simulink library "hapsrav_library"  (R2017a)
settings: Solver=VariableStepAuto  StartTime=0.0  StopTime=10.0  RelTol=1e-3
values from neighbouring files (symbols this model uses):
  absorb_h = 0:100:40000    [EnergySim.m]
  Adisk = pi * v.R_prop^2    [EnergySim.m]
  alpha_h = absorb_h    [EnergySim.m]
  aoa_data = zeros(n_cl, n)    [EnergySim.m]
  cl_bp = linspace(min_cl, max_cl,n_cl)    [EnergySim.m]
  D = [1       -.0065      288.15          0                   101325 ... (first row only)    [EnergySim.m]    (also in msn_params.m = sqrt((from_x - to_x)^2 + (from_y - to_y)^2); solar_vector.m = time.day + ut_time)
  d2r = pi / 180    (= 0.0174532925199)    [EnergySim.m]    (also in example1.m; example2.m; example3.m; example4.m)
  d_init = sqrt(dx*dx + dy*dy)    [EnergySim.m]    (also in msn_init.m)
  dchi0 = atan2(sin(dchi0), cos(dchi0))    [EnergySim.m]    (also in msn_init.m)
  dT = 0.5    [EnergySim.m]
  dT_fixed = 0.5    [EnergySim.m]
  dT_trig = 30    [EnergySim.m]
  earth_rho = 6378137.0    (= 6378137)    [EnergySim.m]
  fp = solarFP(p.orbit_rho, p.min_axis, p.orbit_dir, ic.x_ctr, ic.y_ctr, sun_az_0)    [EnergySim.m]    (also in load_fp.m = gid_tc(msn_idx).fp; solarFP.m = [1	6	2	nul eul 0	0	0	0	1	0)
  fp_coords = [x_entry y_entry]    [msn_params.m]
  fp_courses = [chi_adj nxt_chi dchi]    [msn_params.m]
  g = 9.80665    [EnergySim.m]
  Gsolar = 1367    [EnergySim.m]
  k = k+1    (= 5)    [EnergySim.m]
  K = D(:,2)    [EnergySim.m]
  lat_init = ic.lat_init_deg * obj.d2r    [EnergySim.m]
  M = time.month    [solar_vector.m]
  max_cl = max(cl_data(:))    [EnergySim.m]
  min_cl = min(cl_data(:))    [EnergySim.m]
  ND2 = load(fullfile(pwd,'nd2_data.mat'))    [EnergySim.m]    (also in nd2_data.mat = [0.0999999999999 0.200000000001 0.3 0.4 0.499999999998 0.700)
  next_init = fp(init_wp, 3)    [EnergySim.m]    (also in msn_init.m)
  pE_init = ic.pE_init    [EnergySim.m]
  pN_init = ic.pN_init    [EnergySim.m]
  r2d = 180 / pi    (= 57.2957795131)    [EnergySim.m]    (also in example1.m; example2.m; example3.m; example4.m)
  rho_SL = 1.225    [EnergySim.m]
  S = 110.4    [EnergySim.m]
  thr_lo_lim = 0.0    (= 0)    [EnergySim.m]
  time_init = struct('year', time.year, 'month', time.month,                  'day', time.day, 'hour', time.hour, 'min', time.min,                  'UTC', time.UTC)    [EnergySim.m]
  to_init = fp(init_wp, 1)    [EnergySim.m]    (also in msn_init.m)
  vgnd_init = sqrt(Vg)    [EnergySim.m]
  vtas_init = veas_init * sqrt(rho_sl/rho_alt)    [EnergySim.m]
  w_alt = 2.0 * w_alt    [EnergySim.m]
  w_xtrack = 2.0 * w_xtrack    [EnergySim.m]
undefined symbols (not defined in the file or in its folder): alpha, alpha_bp, alpha_circ, alt0_rate_init, alt_bp, alt_cmd_mode, alt_init, alt_lim_h, alt_lim_l, alt_rt_lim_periodic, cd_data, charge_eff, chi0_rate_init, chi_cmd_mode, chi_inf, chi_init, cl_data, discharge_eff, DiscIntNeverNeededParam, E_batt_max, E_init, Earth, enableFuzzyLogic, entry_init, epsln, epsln_circ, exit_init, f8_azimuth_offset, fig_eight_time, fp0, fp_coords0, fp_courses0, gamma_lim, hold_time, k_c, K_circ, lat_init_deg, lon_init_deg, max_alpha_bp, max_alt_bp, min_alpha_bp, min_alt_bp, min_axis, motor_eff, mppt_eff, num_motors, orb_dir_init, orb_len_init, orbit_dir, orbit_rho, P_acc, panel_eff, panel_vecs, phi_0, phi_lim, phi_lim_alt, phi_lim_alt_max, phi_lim_alt_min, phi_rt_lim, prop_eff_scale ... (+39)
libraries: simulink x59, hapsrav_library x9, fuzblock x3, atmospheric_library x1, aerolibtransform2 x1
(part 4 of 6)

== system hapsrav_library/hapsrav_main/Kinematic 6DOF/Aero/CL vs AoA/alpha RLUT ==
  alt : Inport
  CL : Inport  Port=2
  0 <= Alt < 20574 : Subsystem  Commented=on  TreatAsAtomicUnit=on
  0 <= Alt <= 24575 : Saturate  UpperLimit=max_alt_bp  LowerLimit=min_alt_bp
  0.73 <= CL <= 1.43 : Saturate  UpperLimit=max_cl  LowerLimit=min_cl
  20574 <= Alt < 21908 : Subsystem  Commented=on  TreatAsAtomicUnit=on
  21908 <= Alt < 23241 : Subsystem  Commented=on  TreatAsAtomicUnit=on
  23241 <= Alt < 24575 : Subsystem  Commented=on  TreatAsAtomicUnit=on
  AoA LUT : Lookup_n-D  BreakpointsForDimension1=cl_bp  BreakpointsForDimension2=alt_bp  IndexSearchMethod=Linear search  BeginIndexSearchUsingPreviousIndexResult=on  Table=aoa_data  ExtrapMethod=Clip  RemoveProtectionInput=on  UseLastTableValue=on  InternalRulePriority=Speed  RndMeth=Simplest  InputSameDT=on
  From{,1..2,4,6} (5 alike) : From  Commented=on  GotoTag=alt
  From{3,5,7..8} (4 alike) : From  Commented=on  GotoTag=CL
  Interval Test : simulink/Logic and Bit Operations/Interval Test  Commented=on  IntervalClosedRight=off  uplimit=alt_bp(2)  IntervalClosedLeft=on  lowlimit=alt_bp(1)  OutDataTypeStr=boolean
  Interval Test1 : simulink/Logic and Bit Operations/Interval Test  Commented=on  IntervalClosedRight=off  uplimit=alt_bp(3)  IntervalClosedLeft=on  lowlimit=alt_bp(2)  OutDataTypeStr=boolean
  Interval Test2 : simulink/Logic and Bit Operations/Interval Test  Commented=on  IntervalClosedRight=off  uplimit=alt_bp(4)  IntervalClosedLeft=on  lowlimit=alt_bp(3)  OutDataTypeStr=boolean
  Interval Test3 : simulink/Logic and Bit Operations/Interval Test  Commented=on  IntervalClosedRight=on  uplimit=alt_bp(5)  IntervalClosedLeft=on  lowlimit=alt_bp(4)  OutDataTypeStr=boolean
  Merge : Merge  Commented=on  Inputs=4
  alpha_rad : Outport
  wires:
  0.73 <= CL <= 1.43/1 -> [CL]
  0 <= Alt <= 24575/1 -> [alt]
  From1/1 -> Interval Test/1, Interval Test3/1, Interval Test2/1, Interval Test1/1
  20574 <= Alt < 21908/1(alpha) -> Merge/2
  alt/1 -> 0 <= Alt <= 24575/1
  From8/1 -> 0 <= Alt < 20574/1(CL)
  From3/1 -> 20574 <= Alt < 21908/1(CL)
  0 <= Alt < 20574/1(alpha) -> Merge/1
  Interval Test3/1 -> 23241 <= Alt < 24575/Enable
  From2/1 -> 20574 <= Alt < 21908/2(alt)
  CL/1 -> 0.73 <= CL <= 1.43/1
  Interval Test2/1 -> 21908 <= Alt < 23241/Enable
  23241 <= Alt < 24575/1(alpha) -> Merge/4
  From7/1 -> 23241 <= Alt < 24575/1(CL)
  From4/1 -> 21908 <= Alt < 23241/2(alt)
  From5/1 -> 21908 <= Alt < 23241/1(CL)
  From6/1 -> 23241 <= Alt < 24575/2(alt)
  Interval Test/1 -> 0 <= Alt < 20574/Enable
  21908 <= Alt < 23241/1(alpha) -> Merge/3
  From/1 -> 0 <= Alt < 20574/2(alt)
  Interval Test1/1 -> 20574 <= Alt < 21908/Enable
  [CL] -> AoA LUT/1
  [alt] -> AoA LUT/2
  AoA LUT/1 -> alpha_rad/1

== system hapsrav_library/hapsrav_main/Kinematic 6DOF/Navigation/Flat Earth to LLA/Radii of Curvature ==
  lat_rad : Inport
  h : Inport  Port=2
  Divide : Product  Inputs=*/
  Divide1 : Product  Inputs=**
  Divide2 : Product  Inputs=*/
  Gain1 : Gain  Gain=wgs84.e2
  Math Function : Math  Operator=square  SaturateOnIntegerOverflow=on
  Sqrt : Sqrt  SaturateOnIntegerOverflow=on
  Sum : Sum  Inputs=|+-
  Sum1 : Sum  Inputs=+-|
  Sum2 : Sum  Inputs=|++
  Sum3 : Sum  Inputs=|++
  Trigonometric Function : Trigonometry
  href3 : Constant
  href4 : Constant  Value=wgs84.a
  href5 : Constant  Value=wgs84.e2
  href6 : Constant
  R_N : Outport
  R_M : Outport  Port=2
  wires:
  Sum1/1 -> Divide1/2
  href3/1 -> Sum/1
  Gain1/1 -> Sum/2
  Math Function/1 -> Gain1/1
  Sqrt/1 -> [den_0p5]
  href4/1 -> Divide/1
  href6/1 -> Sum1/1
  href5/1 -> Sum1/2
  Divide/1 -> Divide1/1, Sum2/1  "Prime Vert ROC"
  [den_0p5] -> Divide/2
  [den] -> Divide2/2
  Divide1/1 -> Divide2/1
  lat_rad/1 -> Trigonometric Function/1
  Trigonometric Function/1 -> Math Function/1
  Sum/1 -> Sqrt/1, [den]
  h/1 -> [h]
  Sum2/1 -> R_N/1
  [h] -> Sum2/2
  Divide2/1 -> Sum3/1  "Meridian ROC"
  Sum3/1 -> R_M/1
  [h] -> Sum3/2

== system hapsrav_library/hapsrav_main/Kinematic 6DOF/Power Model/Battery and Potential Management/Climb Rate ==
  ClimbMode : Inport
  P_el_out : Inport  Port=2
  P_el_net_cruise : Inport  Port=3
  P_el_net : Inport  Port=4
  Constant4 : Constant  Value=0
  Constant7 : Constant  Value=P_acc*0.001
  Delay1 : Delay  DelayLength=1
  Gain1 : Gain  Gain=-1
  Gain2 : Gain  Gain=1/M
  Gain3 : Gain  Gain=1/g
  Multiport Switch1 : MultiPortSwitch  DataPortOrder=Specify indices  DataPortIndices={-2, -1, 0, 1}
  PID Controller : simulink/Continuous/PID Controller  Controller=PID  TimeDomain=Discrete-time  SampleTime=-1  IntegratorMethod=Forward Euler  FilterMethod=Forward Euler  Form=Parallel  UseFilter=off  ControllerParametersSource=internal  P=1.1  I=0.001  D=0  N=0.1  InitialConditionSource=internal  InitialConditionForIntegrator=0  InitialConditionForFilter=0  ExternalReset=either  LimitOutput=off  UpperSaturationLimit=inf  LowerSaturationLimit=-inf  LinearizeAsGain=off  AntiWindupMode=none  Kb=1  TrackingMode=off  Kt=1  PParamMin=[]  PParamMax=[]  IParamMin=[]  IParamMax=[]  DParamMin=[]  DParamMax=[]  NParamMin=[]  NParamMax=[]  KbParamMin=[]  KbParamMax=[]  KtParamMin=[]  KtParamMax=[]  POutMin=[]  POutMax=[]  IOutMin=[]  IOutMax=[]  DOutMin=[]  DOutMax=[]  NOutMin=[]  NOutMax=[]  KbOutMin=[]  KbOutMax=[]  KtOutMin=[]  KtOutMax=[]  IntegratorOutMin=[]  IntegratorOutMax=[]  FilterOutMin=[]  FilterOutMax=[]  SumOutMin=[]  SumOutMax=[]  SumI1OutMin=[]  SumI1OutMax=[]  SumI2OutMin=[]  SumI2OutMax=[]  SumI3OutMin=[]  SumI3OutMax=[]  SumDOutMin=[]  SumDOutMax=[]  SaturationOutMin=[]  SaturationOutMax=[]  IntegratorContinuousStateAttributes=''  IntegratorStateMustResolveToSignalObject=off  IntegratorRTWStateStorageClass=Auto  FilterContinuousStateAttributes=''  FilterStateMustResolveToSignalObject=off  FilterRTWStateStorageClass=Auto  DifferentiatorICPrevScaledInput=0  DifferentiatorOutMin=[]  DifferentiatorOutMax=[]  InitialConditionSetting=State (most efficient)
  PID Controller1 : simulink/Continuous/PID Controller  Controller=PID  TimeDomain=Discrete-time  SampleTime=-1  IntegratorMethod=Forward Euler  FilterMethod=Forward Euler  Form=Parallel  UseFilter=off  ControllerParametersSource=internal  P=2.5  I=0.001  D=0  N=0.1  InitialConditionSource=internal  InitialConditionForIntegrator=0  InitialConditionForFilter=0  ExternalReset=either  LimitOutput=off  UpperSaturationLimit=inf  LowerSaturationLimit=-inf  LinearizeAsGain=off  AntiWindupMode=none  Kb=1  TrackingMode=off  Kt=1  PParamMin=[]  PParamMax=[]  IParamMin=[]  IParamMax=[]  DParamMin=[]  DParamMax=[]  NParamMin=[]  NParamMax=[]  KbParamMin=[]  KbParamMax=[]  KtParamMin=[]  KtParamMax=[]  POutMin=[]  POutMax=[]  IOutMin=[]  IOutMax=[]  DOutMin=[]  DOutMax=[]  NOutMin=[]  NOutMax=[]  KbOutMin=[]  KbOutMax=[]  KtOutMin=[]  KtOutMax=[]  IntegratorOutMin=[]  IntegratorOutMax=[]  FilterOutMin=[]  FilterOutMax=[]  SumOutMin=[]  SumOutMax=[]  SumI1OutMin=[]  SumI1OutMax=[]  SumI2OutMin=[]  SumI2OutMax=[]  SumI3OutMin=[]  SumI3OutMax=[]  SumDOutMin=[]  SumDOutMax=[]  SaturationOutMin=[]  SaturationOutMax=[]  IntegratorContinuousStateAttributes=''  IntegratorStateMustResolveToSignalObject=off  IntegratorRTWStateStorageClass=Auto  FilterContinuousStateAttributes=''  FilterStateMustResolveToSignalObject=off  FilterRTWStateStorageClass=Auto  DifferentiatorICPrevScaledInput=0  DifferentiatorOutMin=[]  DifferentiatorOutMax=[]  InitialConditionSetting=State (most efficient)
  Saturation : Saturate  UpperLimit=2.08  LowerLimit=-2.08
  Sum3 : Sum  Inputs=|+-
  kW to W : Gain  Gain=1000
  powered_climb_rt : Outport
  wires:
  PID Controller1/1 -> Multiport Switch1/2
  Constant7/1 -> Sum3/2
  P_el_out/1 -> Sum3/1
  Gain1/1 -> PID Controller1/1
  Sum3/1 -> Gain1/1
  PID Controller/1 -> Multiport Switch1/3
  P_el_net_cruise/1 -> PID Controller/1
  Saturation/1 -> powered_climb_rt/1
  Constant4/1 -> Multiport Switch1/4
  P_el_net/1 -> Multiport Switch1/5
  Multiport Switch1/1 -> Delay1/1
  ClimbMode/1 -> Multiport Switch1/1, PID Controller/2, PID Controller1/2
  Gain3/1 -> Saturation/1  "Max Clmb Rt"
  kW to W/1 -> Gain2/1
  Gain2/1 -> Gain3/1
  Delay1/1 -> kW to W/1

== system hapsrav_library/hapsrav_main/Kinematic 6DOF/Power Model/Electric Power In/atmos_absorb_adj ==
  sun_zth : Inport
  altitude : Inport  Port=2
  Trigger : TriggerPort  TriggerType=either  VariantControl=Variant  InitialTriggerSignalState=positive
  Constant : Constant  Value=earth_rho
  Constant1 : Constant  Value=alpha_h
  Constant2 : Constant  Value=absorb_h
  Gain : Gain  Gain=0.001
  Gain1 : Gain  Gain=0.001
  atmospheric adjustment : MATLAB Function  TreatAsAtomicUnit=on
  atmos_adj : Outport
  wires:
  altitude/1 -> Gain/1
  sun_zth/1 -> atmospheric adjustment/2(zth)
  Constant/1 -> Gain1/1
  Gain/1 -> atmospheric adjustment/1(h)  "h (km)"
  Gain1/1 -> atmospheric adjustment/3(earth_rho)
  Constant1/1 -> atmospheric adjustment/4(alpha_h)
  Constant2/1 -> atmospheric adjustment/5(absorb_h)
  atmospheric adjustment/1(rel_power) -> atmos_adj/1

== system hapsrav_library/hapsrav_main/Kinematic 6DOF/Power Model/Electric Power In/projected area ==
  yaw : Inport
  pitch : Inport  Port=2
  roll : Inport  Port=3
  sun : Inport  Port=4
  Projected area : MATLAB Function  TreatAsAtomicUnit=on
  panel directions : Constant  Value=panel_vecs
  projected_area : Outport
  wires:
  yaw/1 -> Projected area/1(y)
  roll/1 -> Projected area/3(r)
  pitch/1 -> Projected area/2(p)
  Projected area/1(proj_area) -> projected_area/1
  panel directions/1 -> Projected area/4(panel_vecs)
  sun/1 -> Projected area/5(sun_vector)

== system hapsrav_library/hapsrav_main/Kinematic 6DOF/Power Model/Electric Power In/solar_dist_adj ==
  jd : Inport
  Trigger : TriggerPort  TriggerType=either  VariantControl=Variant  InitialTriggerSignalState=positive
  2*pi/365.1 : Gain  Gain=0.034
  2*pi/365.25 : Gain  Gain=2*pi/365.25
  Add : Sum
  Constant : Constant
  Cos : Trigonometry  Operator=cos
  dist_adj : Outport
  wires:
  Constant/1 -> Add/1
  2*pi/365.1/1 -> Add/2
  Cos/1 -> 2*pi/365.1/1
  jd/1 -> 2*pi/365.25/1
  2*pi/365.25/1 -> Cos/1
  Add/1 -> dist_adj/1

== system hapsrav_library/hapsrav_main/Kinematic 6DOF/Power Model/Electric Power In/solar_vec_ned ==
  az : Inport
  zth : Inport  Port=2
  Trigger : TriggerPort  TriggerType=either  VariantControl=Variant  InitialTriggerSignalState=positive
  Gain1 : Gain  Gain=d2r
  Gain2 : Gain  Gain=d2r
  Gain3 : Gain  Gain=-1
  Gain4 : Gain  Gain=-1
  Mux1 : Mux  Inputs=3
  Mux2 : Mux  Inputs=3
  Subtract : Sum  Inputs=-+
  Trigonometric Function : Trigonometry
  Trigonometric Function1 : Trigonometry  Operator=cos
  Trigonometric Function2 : Trigonometry
  Trigonometric Function3 : Trigonometry  Operator=cos
  clip when below horizon : Switch  Criteria=u2 > Threshold
  complement : Constant  Value=pi/2
  complement1 : Constant  Value=0
  complement2 : Constant  Value=0
  complement3 : Constant  Value=0
  pow_calc1 : Product
  pow_calc2 : Product
  sun_ned : Outport
  wires:
  Gain2/1 -> Subtract/1
  Gain4/1 -> Mux1/2
  complement3/1 -> Mux2/3
  [c_el] -> pow_calc1/2
  zth/1 -> Gain2/1
  az/1 -> Gain1/1
  Mux2/1 -> clip when below horizon/3
  Gain3/1 -> Mux1/1
  Subtract/1 -> clip when below horizon/2, Trigonometric Function3/1, Trigonometric Function2/1  "el"
  Trigonometric Function1/1 -> [c_az]
  complement2/1 -> Mux2/2
  Trigonometric Function2/1 -> [s_el]
  [s_az] -> pow_calc2/1
  [c_el] -> pow_calc2/2
  [s_el] -> Mux1/3
  complement1/1 -> Mux2/1
  Trigonometric Function3/1 -> [c_el]
  Gain1/1 -> Trigonometric Function1/1, Trigonometric Function/1
  [c_az] -> pow_calc1/1
  clip when below horizon/1 -> sun_ned/1
  Mux1/1 -> clip when below horizon/1
  complement/1 -> Subtract/2
  Trigonometric Function/1 -> [s_az]
  pow_calc2/1 -> Gain4/1
  pow_calc1/1 -> Gain3/1

== system hapsrav_library/hapsrav_main/Kinematic 6DOF/Power Model/Electric Power Out/prop_eff (theoretical max from actuator disk theory, scaled by coeff < 1) (http:////web.mit.edu//16.unified//www//FALL//thermodynamics//notes//node86.html) ==
  thrust : Inport
  qbar : Inport  Port=2
  Add : Sum
  Add1 : Sum
  Constant : Constant
  Constant1 : Constant
  Constant2 : Constant  Value=2
  Divide1 : Product  Inputs=*/
  Divide2 : Product  Inputs=*/
  Sqrt : Sqrt  SaturateOnIntegerOverflow=on
  disk_area : Gain  Gain=Adisk
  num_motors : Gain  Gain=num_motors
  scale_by_const : Gain  Gain=prop_eff_scale
  prop_eff : Outport
  wires:
  Constant2/1 -> Divide2/1
  Divide1/1 -> Add/2
  Divide2/1 -> scale_by_const/1  "theoretical max"
  Constant/1 -> Add/1
  Add/1 -> Sqrt/1
  Add1/1 -> Divide2/2
  Sqrt/1 -> Add1/2
  Constant1/1 -> Add1/1
  scale_by_const/1 -> prop_eff/1
  thrust/1 -> Divide1/1
  disk_area/1 -> num_motors/1
  num_motors/1 -> Divide1/2
  qbar/1 -> disk_area/1

== system hapsrav_library/hapsrav_main/Kinematic 6DOF/Selectable Modes/Trajectory_Optimization/Altitude ==
  altRt_cmd : Inport
  max_clmb_rt : Inport  Port=2
  max_desc_rt : Inport  Port=3
  alt0 : Inport  Port=4
  altRt0 : Inport  Port=5
  idleDesc : Inport  Port=6
  Delay1 : Delay  DelayLength=1  InitialConditionSource=Input port
      settings: InputPortMap=u0,p4
  Discrete-Time Integrator : DiscreteIntegrator  IntegratorMethod=Integration: Trapezoidal  InitialConditionSource=external  InitialConditionSetting=State (most efficient)  SampleTime=-1  ICPrevOutput=DiscIntNeverNeededParam  ICPrevScaledInput=DiscIntNeverNeededParam
  Mux : Mux  Inputs=2
  Scope : Scope
  Sum : Sum  Inputs=|+-
  alt_rate : Subsystem
  u_wn^2 : Gain  Gain=w_alt * w_alt
  alt : Outport
  d1alt : Outport  Port=2
  wires:
  [alt_rate] -> Mux/1
  [cmd] -> Mux/2
  [cmd] -> Sum/1
  altRt_cmd/1 -> [cmd]
  Mux/1 -> Scope/1
  [alt_rate] -> d1alt/1
  max_desc_rt/1 -> alt_rate/2(max_desc_rt)
  idleDesc/1 -> alt_rate/5(idleDesc)
  alt0/1 -> Discrete-Time Integrator/2
  Delay1/1 -> Sum/2
  alt_rate/1(d1alt) -> Discrete-Time Integrator/1, [alt_rate], Delay1/1
  Discrete-Time Integrator/1 -> alt/1
  Sum/1 -> u_wn^2/1
  max_clmb_rt/1 -> alt_rate/1(max_clmb_rt)
  u_wn^2/1 -> alt_rate/3(d2alt)
  altRt0/1 -> [altRt0]
  [altRt0] -> Delay1/2
  [altRt0] -> alt_rate/4(altRt0)

== system hapsrav_library/hapsrav_main/Kinematic 6DOF/Selectable Modes/Trajectory_Optimization/Lat Cmd Filter ==
  roll cmd : Inport
  roll0 : Inport  Port=2
  1/tau : Gain  Gain=0.1
  Delay1 : Delay  DelayLength=1  InitialConditionSource=Input port
      settings: InputPortMap=u0,p4
  Discrete-Time Integrator : DiscreteIntegrator  IntegratorMethod=Integration: Trapezoidal  InitialConditionSource=external  InitialConditionSetting=State (most efficient)  SampleTime=-1  ICPrevOutput=DiscIntNeverNeededParam  ICPrevScaledInput=DiscIntNeverNeededParam
  Sum : Sum  Inputs=|+-
  filt roll cmd : Outport
  wires:
  [roll0] -> Discrete-Time Integrator/2
  [roll0] -> Delay1/2
  roll0/1 -> [roll0]
  Delay1/1 -> Sum/2
  roll cmd/1 -> Sum/1
  Discrete-Time Integrator/1 -> filt roll cmd/1, Delay1/1
  Sum/1 -> 1/tau/1
  1/tau/1 -> Discrete-Time Integrator/1

== system hapsrav_library/hapsrav_main/Kinematic 6DOF/Selectable Modes/Trajectory_Optimization/Roll ==
  filtRollcmd : Inport
  roll0 : Inport  Port=2
  alt : Inport  Port=3
  Vg : Inport  Port=4
  chi0 : Inport  Port=5
  Delay1 : Delay  DelayLength=1  InitialConditionSource=Input port
      settings: InputPortMap=u0,p4
  Saturation Dynamic : simulink/Discontinuities/Saturation Dynamic  OutMin=[]  OutMax=[]  OutDataTypeStr=Inherit: Same as second input  OutDataType=fixdt(1, 16)  OutScaling=2^-10  DoSatur=off
  Sum : Sum  Inputs=|+-
  a : Gain  Gain=-1
  phi_lim LUT : Lookup_n-D  NumberOfTableDimensions=1  BreakpointsForDimension1=phi_lim_alt  Table=phi_lim  ExtrapMethod=Clip  DiagnosticForOutOfRangeInput=Error  RemoveProtectionInput=on  UseLastTableValue=on  InternalRulePriority=Speed  RndMeth=Simplest  InputSameDT=on
  phi_rt_lim LUT : Lookup_n-D  NumberOfTableDimensions=1  BreakpointsForDimension1=phi_lim_alt  Table=phi_rt_lim  ExtrapMethod=Clip  DiagnosticForOutOfRangeInput=Error  RemoveProtectionInput=on  UseLastTableValue=on  InternalRulePriority=Speed  RndMeth=Simplest  InputSameDT=on
  roll_angle : Subsystem
  u_wn^2 : Gain  Gain=w_xtrack * w_xtrack
  roll : Outport
  chi : Outport  Port=2
  wires:
  roll_angle/1(chi) -> chi/1
  chi0/1 -> roll_angle/5(chi0)
  Vg/1 -> roll_angle/4(Vg)
  u_wn^2/1 -> Saturation Dynamic/2
  filtRollcmd/1 -> Sum/1
  Sum/1 -> u_wn^2/1
  roll_angle/2(roll) -> Delay1/1, roll/1
  Delay1/1 -> Sum/2
  roll0/1 -> roll_angle/3(roll0), [roll0]
  [roll0] -> Delay1/2
  phi_lim LUT/1 -> [phi_lim]
  phi_rt_lim LUT/1 -> [phi_rt_lim]
  alt/1 -> phi_rt_lim LUT/1, phi_lim LUT/1
  [phi_lim] -> roll_angle/1(roll_lim)
  [phi_rt_lim] -> Saturation Dynamic/1
  [phi_rt_lim] -> a/1
  a/1 -> Saturation Dynamic/3
  Saturation Dynamic/1 -> roll_angle/2(d1roll)

== system hapsrav_library/hapsrav_main/Kinematic 6DOF/Selectable Modes/Trajectory_Optimization/Vert Cmd Filter ==
  hdot_cmd : Inport
  altRt0 : Inport  Port=2
  uplim : Inport  Port=3
  lolim : Inport  Port=4
  1/tau : Gain  Gain=0.1
  Constant : Constant  Value=dT
  Delay1 : Delay  DelayLength=1  InitialConditionSource=Input port
      settings: InputPortMap=u0,p4
  Delay2 : Delay  DelayLength=1  InitialConditionSource=Input port
      settings: InputPortMap=u0,p4
  Limited Integration : MATLAB Function  TreatAsAtomicUnit=on
  Scope : Scope
  Sum : Sum  Inputs=|+-
  filt hdot cmd : Outport
  wires:
  lolim/1 -> Limited Integration/4(lolim)
  uplim/1 -> Limited Integration/3(uplim)
  Constant/1 -> Limited Integration/2(T)
  Delay2/1 -> Limited Integration/5(x0)
  Limited Integration/2(x1) -> Delay2/1
  [altRt0] -> Delay2/2
  Delay1/1 -> Sum/2
  [altRt0] -> Delay1/2
  altRt0/1 -> [altRt0]
  hdot_cmd/1 -> Sum/1
  Limited Integration/1(y0) -> filt hdot cmd/1, Scope/1, Delay1/1
  Sum/1 -> 1/tau/1
  1/tau/1 -> Limited Integration/1(u)

== system hapsrav_library/hapsrav_main/Kinematic 6DOF/Selectable Modes/Waypoint_Navigation/Altitude ==
  alt_cmd : Inport
  alt0 : Inport  Port=2
  max_clmb_rt : Inport  Port=3
  max_desc_rt : Inport  Port=4
  alt_rt_init : Inport  Port=5
  idleDesc : Inport  Port=6
  2*z*wn : Gain  Gain=2*z_alt*w_alt
  Delay1 : Delay  DelayLength=1  InitialConditionSource=Input port
      settings: InputPortMap=u0,p4
  Discrete-Time Integrator : DiscreteIntegrator  IntegratorMethod=Integration: Trapezoidal  InitialConditionSource=external  InitialConditionSetting=State (most efficient)  SampleTime=-1  ICPrevOutput=DiscIntNeverNeededParam  ICPrevScaledInput=DiscIntNeverNeededParam
  Sum : Sum  Inputs=|+-
  Sum2 : Sum  Inputs=++|
  alt_rate : Subsystem
  u_wn^2 : Gain  Gain=w_alt * w_alt
  wn*wn : Gain  Gain=w_alt*w_alt
  x0_wn^2 : Gain  Gain=w_alt * w_alt
  alt : Outport
  d1alt : Outport  Port=2
  wires:
  idleDesc/1 -> alt_rate/5(idleDesc)
  alt_rt_init/1 -> alt_rate/4(altRt0)
  Sum/1 -> alt_rate/3(d2alt)
  alt_cmd/1 -> u_wn^2/1
  Discrete-Time Integrator/1 -> wn*wn/1, alt/1
  u_wn^2/1 -> Sum/1
  alt_rate/1(d1alt) -> d1alt/1, 2*z*wn/1, Discrete-Time Integrator/1
  max_desc_rt/1 -> alt_rate/2(max_desc_rt)
  wn*wn/1 -> Sum2/2
  2*z*wn/1 -> Sum2/1
  Sum2/1 -> Delay1/1
  Delay1/1 -> Sum/2
  x0_wn^2/1 -> Delay1/2
  alt0/1 -> [alt0]
  [alt0] -> Discrete-Time Integrator/2
  [alt0] -> x0_wn^2/1
  max_clmb_rt/1 -> alt_rate/1(max_clmb_rt)

== system hapsrav_library/hapsrav_main/Kinematic 6DOF/Selectable Modes/Waypoint_Navigation/Course ==
  Vg : Inport
  alt : Inport  Port=2
  chi_cmd : Inport  Port=3
  chi0 : Inport  Port=4
  d1Vg : Inport  Port=5
  2*z/wn : Gain  Gain=2*z_xtrack/w_xtrack
  Circular Integration : Subsystem
  Delay1 : Delay  DelayLength=1  InitialConditionSource=Input port
      settings: InputPortMap=u0,p4
  MATLAB Function2 : MATLAB Function  TreatAsAtomicUnit=on
  Rate Limits : Subsystem
  Sum2 : Sum  Inputs=++|
  Wrap +/- pi : Subsystem
  chi_dot : Subsystem
  wn^2 : Gain  Gain=w_xtrack * w_xtrack
  phi : Outport
  chi : Outport  Port=2
  wires:
  [chi0] -> Circular Integration/2(x0)
  Circular Integration/1(y) -> Sum2/2, chi/1
  Wrap +/- pi/1(ang_pi) -> MATLAB Function2/1(ref)
  MATLAB Function2/1(circ_err) -> wn^2/1
  chi_cmd/1 -> Wrap +/- pi/1(ang)
  wn^2/1 -> Rate Limits/3(d2chi)
  Delay1/1 -> MATLAB Function2/2(posn)
  chi_dot/2(d1chi) -> 2*z/wn/1, Circular Integration/1(u)
  Rate Limits/2(d2chi_lim) -> chi_dot/3(d2chi)
  [Vg] -> Rate Limits/1(Vg)
  [Vg] -> chi_dot/1(Vg)
  alt/1 -> Rate Limits/2(alt)
  Rate Limits/1(phi_lim) -> chi_dot/2(phi_lim)
  2*z/wn/1 -> Sum2/1
  Sum2/1 -> Delay1/1
  [chi0] -> Delay1/2
  chi0/1 -> [chi0]
  Vg/1 -> [Vg]
  d1Vg/1 -> Rate Limits/4(d1Vg)
  chi_dot/1(phi) -> phi/1

== system hapsrav_library/hapsrav_main/Kinematic 6DOF/Selectable Modes/Waypoint_Navigation/Lat Cmd Filter ==
  chi cmd : Inport
  chi_init : Inport  Port=2
  Compare To Constant3 : simulink/Logic and Bit Operations/Compare To Constant  relop=>=  const=4  OutDataTypeStr=boolean
  Constant : Constant  Value=chi_cmd_mode
  Filtered Command : Subsystem  TreatAsAtomicUnit=on
  Logical Operator : Logic  Operator=NOT  Inputs=1  AllPortsSameDT=off  OutDataTypeStr=boolean
  Merge : Merge
  Unfiltered Command : Subsystem  TreatAsAtomicUnit=on
  filt chi cmd : Outport
  wires:
  Merge/1 -> filt chi cmd/1
  Filtered Command/1(filt chi cmd) -> Merge/2
  Unfiltered Command/1(cmdFilt) -> Merge/1
  Logical Operator/1 -> Filtered Command/Enable
  chi_init/1 -> Filtered Command/2(chi_init)
  chi cmd/1 -> Filtered Command/1(chi cmd), Unfiltered Command/1(cmd)
  Compare To Constant3/1 -> Logical Operator/1, Unfiltered Command/Enable
  Constant/1 -> Compare To Constant3/1

== system hapsrav_library/hapsrav_main/Kinematic 6DOF/Selectable Modes/Waypoint_Navigation/Vert Cmd Filter ==
  alt cmd : Inport
  alt_init : Inport  Port=2
  max_clmb_rt : Inport  Port=3
  max_desc_rt : Inport  Port=4
  1/tau : Gain  Gain=0.1
  Delay1 : Delay  DelayLength=1  InitialConditionSource=Input port
      settings: InputPortMap=u0,p4
  Discrete-Time Integrator : DiscreteIntegrator  IntegratorMethod=Integration: Trapezoidal  InitialConditionSource=external  InitialConditionSetting=State (most efficient)  SampleTime=-1  ICPrevOutput=DiscIntNeverNeededParam  ICPrevScaledInput=DiscIntNeverNeededParam
  Saturation Dynamic : simulink/Discontinuities/Saturation Dynamic  OutMin=[]  OutMax=[]  OutDataTypeStr=Inherit: Same as second input  OutDataType=fixdt(1, 16)  OutScaling=2^-10  DoSatur=off
  Sum : Sum  Inputs=|+-
  filt alt cmd : Outport
  wires:
  max_desc_rt/1 -> Saturation Dynamic/3
  max_clmb_rt/1 -> Saturation Dynamic/1
  Saturation Dynamic/1 -> Discrete-Time Integrator/1
  1/tau/1 -> Saturation Dynamic/2
  Sum/1 -> 1/tau/1
  Discrete-Time Integrator/1 -> Delay1/1, filt alt cmd/1
  alt cmd/1 -> Sum/1
  alt_init/1 -> [alt_init]
  [alt_init] -> Delay1/2
  Delay1/1 -> Sum/2
  [alt_init] -> Discrete-Time Integrator/2

== system hapsrav_library/Cmd - Parametric/Chi Cmd/Flight Plan/Mission Command/Entry Mode/Desired Course ==
  leg_crs : Inport
  xtrack : Inport  Port=2
  Enable : EnablePort
  Desired Course : Subsystem
  Sum : Sum  Inputs=|++
  chi_d : Outport
  wires:
  leg_crs/1 -> Sum/1
  xtrack/1 -> Desired Course/1(xtrack)
  Sum/1 -> chi_d/1
  Desired Course/1(chi_d) -> Sum/2

== system hapsrav_library/Cmd - Parametric/Chi Cmd/Flight Plan/Mission Command/Entry Mode/Desired Course1 ==
  leg_state : Inport
  av_posn : Inport  Port=2
  Enable : EnablePort
  Bus Selector : BusSelector  OutputSignals=leg_coords.to_x,leg_coords.to_y
  Demux1 : Demux
  Sum1 : Sum  Inputs=|+-
  Sum2 : Sum  Inputs=|+-
  Terminator : Terminator
  Terminator1 : Terminator
  Trigonometric Function : Trigonometry  Operator=atan2
  chi_d : Outport
  wires:
  Trigonometric Function/1 -> chi_d/1
  Sum2/1 -> Trigonometric Function/2
  Sum1/1 -> Trigonometric Function/1
  [av_x] -> Sum2/2
  [x1] -> Sum2/1
  [av_y] -> Sum1/2
  [y1] -> Sum1/1
  Bus Selector/2 -> [y1]  "<to_y>"
  Bus Selector/1 -> [x1]  "<to_x>"
  Demux1/4 -> Terminator1/1
  Demux1/3 -> Terminator/1
  av_posn/1 -> Demux1/1
  Demux1/2 -> [av_y]
  Demux1/1 -> [av_x]
  leg_state/1 -> Bus Selector/1

== system hapsrav_library/Cmd - Parametric/Chi Cmd/Flight Plan/Mission Command/Entry Mode/xtrack Error ==
  leg_state : Inport
  av_posn : Inport  Port=2
  Bus Selector : BusSelector  OutputSignals=leg_coords.to_x,leg_coords.to_y,crs_state.leg_crs
  Compare To Constant : simulink/Logic and Bit Operations/Compare To Constant  relop=<=  const=10  OutDataTypeStr=boolean
  Demux1 : Demux
  Distance : Subsystem  TreatAsAtomicUnit=on
  MATLAB Function : MATLAB Function  TreatAsAtomicUnit=on
  Product{,1..3} (4 alike) : Product
  Sum{,1..2,4} (4 alike) : Sum  Inputs=|+-
  Sum3 : Sum  Inputs=|++
  leg_crs : Outport
  xtrk : Outport  Port=2
  collocated : Outport  Port=3
  wires:
  Compare To Constant/1 -> collocated/1
  av_posn/1 -> Demux1/1
  Demux1/4 -> [y2]
  Demux1/3 -> [x2]
  Demux1/2 -> [av_y]
  Demux1/1 -> [av_x]
  Bus Selector/3 -> leg_crs/1  "<leg_crs>"
  Distance/1(Dist) -> MATLAB Function/2(den), Compare To Constant/1
  [y2] -> Distance/4(from_y)
  [y1] -> Distance/3(to_y)
  [x2] -> Distance/2(from_x)
  [x1] -> Distance/1(to_x)
  Bus Selector/2 -> [y1]  "<to_y>"
  Bus Selector/1 -> [x1]  "<to_x>"
  MATLAB Function/1(xtrack) -> xtrk/1
  Sum4/1 -> MATLAB Function/1(num)
  Sum2/1 -> Sum3/1
  Product2/1 -> Sum3/2
  Product/1 -> Sum2/1
  [av_x] -> Product/2
  [y2] -> Sum1/1
  [av_y] -> Product1/2
  [x1] -> Sum/2
  leg_state/1 -> Bus Selector/1
  [x1] -> Product3/2
  [y2] -> Product3/1
  [x2] -> Sum/1
  [dx] -> Product1/1
  [dy] -> Product/1
  Sum3/1 -> Sum4/1
  [x2] -> Product2/1
  Product1/1 -> Sum2/2
  Sum1/1 -> [dy]
  [y1] -> Sum1/2
  Sum/1 -> [dx]
  Product3/1 -> Sum4/2
  [y1] -> Product2/2

== system hapsrav_library/Cmd - Parametric/Chi Cmd/Flight Plan/Mission Command/Not Entry Mode/Circular Pattern Holding ==
  note: % k_c needs to be scheduled with Vgnd
  av_state : Inport
  orbit_state : Inport  Port=2
  Enable : EnablePort  StatesWhenEnabling=reset
  Bus Selector : BusSelector  OutputSignals=av_posn,av_course,av_gndspeed
  Bus Selector1 : BusSelector  OutputSignals=x_ctr,y_ctr,orbit_dir,orbit_rho
  Constant12 : Constant  Value=k_c
  Constant2 : Constant  Value=epsln_circ
  Constant4 : Constant  Value=alpha_circ
  Constant5 : Constant  Value=K_circ
  Demux1 : Demux
  MATLAB Function1 : MATLAB Function  TreatAsAtomicUnit=on
  MATLAB Function3 : MATLAB Function  TreatAsAtomicUnit=on
  Mux2 : Mux  Inputs=2
  Sum : Sum  Inputs=|+-
  Sweep Angle : Subsystem
  Terminator : Terminator
  chi_cmd : Outport
  chi_d : Outport  Port=2
  xtrack : Outport  Port=3
  sweep : Outport  Port=4
  wires:
  Sweep Angle/1(swept_angle) -> sweep/1
  [x_ctr] -> Sweep Angle/4(x_ctr)
  [av_x] -> Sweep Angle/3(av_x)
  [y_ctr] -> Sweep Angle/2(y_ctr)
  [av_y] -> Sweep Angle/1(av_y)
  [orbit_dir] -> MATLAB Function1/5(orbit_dir)
  Bus Selector1/4 -> [orbit_rho]  "<orbit_rho>"
  Bus Selector1/3 -> [orbit_dir]  "<orbit_dir>"
  Bus Selector1/2 -> [y_ctr]  "<y_ctr>"
  Bus Selector1/1 -> [x_ctr]  "<x_ctr>"
  [y_ctr] -> MATLAB Function1/4(y_c)
  orbit_state/1 -> Bus Selector1/1
  [chi_d] -> chi_d/1
  [av_y] -> MATLAB Function1/2(av_y)
  Demux1/2 -> [av_y]
  Demux1/1 -> [av_x]
  Mux2/1 -> Terminator/1
  Demux1/4 -> Mux2/2
  Demux1/3 -> Mux2/1
  Sum/1 -> xtrack/1
  [orbit_rho] -> Sum/2
  [dist] -> Sum/1
  [orbit_rho] -> MATLAB Function1/6(r_c)
  Constant4/1 -> MATLAB Function3/7(alpha)
  [x_ctr] -> MATLAB Function1/3(x_c)
  [Vg] -> MATLAB Function3/6(Vg)
  [chi] -> MATLAB Function3/1(chi)
  [av_x] -> MATLAB Function1/1(av_x)
  Bus Selector/3 -> [Vg]  "<av_gndspeed>"
  Bus Selector/2 -> [chi]  "<av_course>"
  Bus Selector/1 -> Demux1/1  "<av_posn>"
  av_state/1 -> Bus Selector/1
  Constant2/1 -> MATLAB Function3/8(e)
  Constant5/1 -> MATLAB Function3/9(K)
  MATLAB Function1/3(beta) -> [beta]
  MATLAB Function3/1(chi_cmd) -> chi_cmd/1
  [beta] -> MATLAB Function3/5(beta)
  [chi_d] -> MATLAB Function3/4(chi_d)
  [rel_ang] -> MATLAB Function3/3(g)
  [dist] -> MATLAB Function3/2(d)
  MATLAB Function1/2(g) -> [rel_ang]
  MATLAB Function1/1(d) -> [dist]
  MATLAB Function1/4(chi_d) -> [chi_d]
  Constant12/1 -> MATLAB Function1/7(k_c)

== system hapsrav_library/Cmd - Parametric/Chi Cmd/Flight Plan/Mission Command/Not Entry Mode/Linear Following ==
  leg_state : Inport
  av_state : Inport  Port=2
  Enable : EnablePort
  Bus Selector2 : BusSelector  OutputSignals=leg_coords,crs_state.leg_crs
  Constant : Constant  Value=0
  Path Following : Subsystem
  chi_cmd : Outport
  chi_d : Outport  Port=2
  xtrack : Outport  Port=3
  sweep : Outport  Port=4
  wires:
  Constant/1 -> sweep/1
  av_state/1 -> Path Following/3(av_state)
  [leg_crs] -> Path Following/2(leg_crs)
  Bus Selector2/2 -> [leg_crs]  "<leg_crs>"
  Bus Selector2/1 -> [leg_coords]  "<leg_coords>"
  leg_state/1 -> Bus Selector2/1
  [leg_coords] -> Path Following/1(leg_coords)
  Path Following/3(xtrack) -> xtrack/1
  Path Following/2(chi_d) -> chi_d/1
  Path Following/1(chi_cmd) -> chi_cmd/1

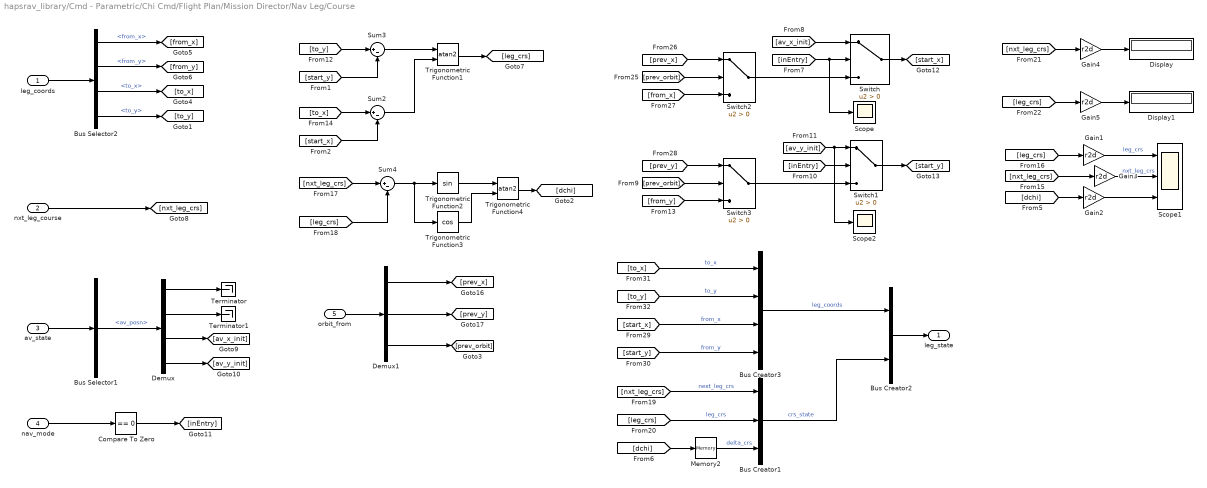
== system hapsrav_library/Cmd - Parametric/Chi Cmd/Flight Plan/Mission Director/Nav Leg/Course ==
  leg_coords : Inport
  nxt_leg_course : Inport  Port=2
  av_state : Inport  Port=3
  nav_mode : Inport  Port=4
  orbit_from : Inport  Port=5
  Bus Creator1 : BusCreator  Inputs='next_leg_crs','leg_crs','delta_crs'
  Bus Creator2 : BusCreator  Inputs='leg_coords','crs_state'
  Bus Creator3 : BusCreator  Inputs='to_x','to_y','from_x','from_y'
  Bus Selector1 : BusSelector  OutputSignals=av_posn
  Bus Selector2 : BusSelector  OutputSignals=from_x,from_y,to_x,to_y
  Compare To Zero : simulink/Logic and Bit Operations/Compare To Zero  relop===  OutDataTypeStr=boolean
  Demux : Demux
  Demux1 : Demux  Outputs=3
  Display : Display
  Display1 : Display
  Gain{1..5} (5 alike) : Gain  Gain=r2d
  Memory2 : Memory  X0=dchi0
  Scope : Scope
  Scope1 : Scope  NumInputPorts=3
  Scope2 : Scope
  Sum2 : Sum  Inputs=|+-
  Sum3 : Sum  Inputs=|+-
  Sum4 : Sum  Inputs=|+-
  Switch{,1..3} (4 alike) : Switch  Criteria=u2 > Threshold
  Terminator : Terminator
  Terminator1 : Terminator
  Trigonometric Function1 : Trigonometry  Operator=atan2
  Trigonometric Function2 : Trigonometry
  Trigonometric Function3 : Trigonometry  Operator=cos
  Trigonometric Function4 : Trigonometry  Operator=atan2
  leg_state : Outport
  wires:
  [start_y] -> Bus Creator3/4  "from_y"
  [start_x] -> Bus Creator3/3  "from_x"
  [to_x] -> Bus Creator3/1  "to_x"
  [to_y] -> Bus Creator3/2  "to_y"
  [prev_y] -> Switch3/1
  [prev_orbit] -> Switch3/2
  [from_y] -> Switch3/3
  Switch3/1 -> Switch1/3
  Switch2/1 -> Switch/3
  [from_x] -> Switch2/3
  [prev_x] -> Switch2/1
  [prev_orbit] -> Switch2/2
  Demux1/2 -> [prev_y]
  Demux1/1 -> [prev_x]
  Demux1/3 -> [prev_orbit]
  orbit_from/1 -> Demux1/1
  [dchi] -> Memory2/1
  Memory2/1 -> Bus Creator1/3  "delta_crs"
  [leg_crs] -> Gain5/1
  Gain5/1 -> Display1/1
  [nxt_leg_crs] -> Gain4/1
  Gain4/1 -> Display/1
  [dchi] -> Gain2/1
  Trigonometric Function4/1 -> [dchi]
  Bus Creator2/1 -> leg_state/1
  nxt_leg_course/1 -> [nxt_leg_crs]
  Bus Creator3/1 -> Bus Creator2/1  "leg_coords"
  Bus Selector2/4 -> [to_y]  "<to_y>"
  Bus Selector2/3 -> [to_x]  "<to_x>"
  Bus Selector2/2 -> [from_y]  "<from_y>"
  Bus Selector2/1 -> [from_x]  "<from_x>"
  leg_coords/1 -> Bus Selector2/1
  Gain3/1 -> Scope1/2  "nxt_leg_crs"
  Gain1/1 -> Scope1/1  "leg_crs"
  [nxt_leg_crs] -> Bus Creator1/1  "next_leg_crs"
  [leg_crs] -> Bus Creator1/2  "leg_crs"
  Bus Creator1/1 -> Bus Creator2/2  "crs_state"
  Gain2/1 -> Scope1/3
  Trigonometric Function3/1 -> Trigonometric Function4/2
  Trigonometric Function2/1 -> Trigonometric Function4/1
  Sum4/1 -> Trigonometric Function2/1, Trigonometric Function3/1
  [leg_crs] -> Sum4/2
  [nxt_leg_crs] -> Sum4/1
  [leg_crs] -> Gain1/1
  [nxt_leg_crs] -> Gain3/1
  Trigonometric Function1/1 -> [leg_crs]
  Demux/2 -> Terminator1/1
  Demux/1 -> Terminator/1
  Switch1/1 -> [start_y]
  [av_y_init] -> Switch1/1, Scope2/1
  [inEntry] -> Switch1/2
  Switch/1 -> [start_x]
  [av_x_init] -> Switch/1
  [inEntry] -> Switch/2, Scope/1
  Compare To Zero/1 -> [inEntry]
  nav_mode/1 -> Compare To Zero/1
  Demux/4 -> [av_y_init]
  Demux/3 -> [av_x_init]
  Bus Selector1/1 -> Demux/1  "<av_posn>"
  av_state/1 -> Bus Selector1/1
  [start_x] -> Sum2/2
  [start_y] -> Sum3/2
  [to_x] -> Sum2/1
  Sum2/1 -> Trigonometric Function1/2
  [to_y] -> Sum3/1
  Sum3/1 -> Trigonometric Function1/1

== system hapsrav_library/Cmd - Parametric/Chi Cmd/Flight Plan/Mission Director/Nav Leg/Flight Plan ==
  nav_md : Inport
  sol_az : Inport  Port=2  OutDataTypeStr=double  PortDimensions=1
  Compare To Constant : simulink/Logic and Bit Operations/Compare To Constant  relop===  const=1  OutDataTypeStr=boolean
  Realtime FP : Subsystem
  Scope1 : Scope
  fp : Outport  PortDimensions=[6,11]
  fp_courses : Outport  Port=2  PortDimensions=[6,3]
  fp_coords : Outport  Port=3  PortDimensions=[6,2]
  wires:
  Realtime FP/3(fp_coords) -> fp_coords/1
  Realtime FP/2(fp_courses) -> fp_courses/1
  sol_az/1 -> Realtime FP/1(sol_az)
  Realtime FP/1(fp) -> fp/1
  Compare To Constant/1 -> Realtime FP/Enable, Scope1/1
  nav_md/1 -> Compare To Constant/1

== system hapsrav_library/Cmd - Parametric/Chi Cmd/Flight Plan/Mission Director/Nav Leg/Mission Plan ==
  WP to : Inport
  fp : Inport  Port=2
  Assignment : Assignment  DiagnosticForDimensions=Warning  IndexOptions=Index vector (port)  Indices=1  OutputSizes=1
  Constant : Constant  Value=sel_vec
  Constant1 : Constant
  Gain : Gain  Commented=on  Gain=fp  Multiplication=Matrix(u*K)
  Product : Product  Multiplication=Matrix(*)
  Reshape : Reshape  OutputDimensionality=Row vector (2-D)
  WP params : Outport
  wires:
  fp/1 -> Product/2
  Reshape/1 -> Product/1
  Assignment/1 -> Reshape/1
  Product/1 -> WP params/1
  Constant1/1 -> Assignment/2
  WP to/1 -> Assignment/3
  Constant/1 -> Assignment/1

== system hapsrav_library/Cmd - Parametric/Chi Cmd/Flight Plan/Mission Director/Nav Leg/Mission Plan1 ==
  WP to : Inport
  fp : Inport  Port=2
  Assignment : Assignment  DiagnosticForDimensions=Warning  IndexOptions=Index vector (port)  Indices=1  OutputSizes=1
  Constant : Constant  Value=sel_vec
  Constant1 : Constant
  Demux : Demux  Outputs=11
  Gain : Gain  Commented=on  Gain=fp  Multiplication=Matrix(u*K)
  Mux : Mux  Inputs=3
  Product : Product  Multiplication=Matrix(*)
  Reshape : Reshape  OutputDimensionality=Row vector (2-D)
  Terminator{,1..2,5..9} (8 alike) : Terminator
  orbit_from : Outport
  wires:
  Product/1 -> Demux/1
  fp/1 -> Product/2
  Reshape/1 -> Product/1
  Assignment/1 -> Reshape/1
  Mux/1 -> orbit_from/1
  Demux/6 -> Mux/3  "orbit_flag"
  Demux/11 -> Terminator9/1
  Demux/10 -> Terminator8/1
  Demux/9 -> Terminator7/1
  Demux/8 -> Terminator6/1
  Demux/7 -> Terminator5/1
  Demux/5 -> Mux/2  "to_y"
  Demux/4 -> Mux/1  "to_x"
  Demux/3 -> Terminator2/1
  Demux/2 -> Terminator1/1
  Demux/1 -> Terminator/1
  Constant/1 -> Assignment/1
  WP to/1 -> Assignment/3
  Constant1/1 -> Assignment/2

== system hapsrav_library/Cmd - Parametric/Chi Cmd/Flight Plan/Mission Director/Nav Leg/WP Coords ==
  to_wp : Inport
  from_wp : Inport  Port=2
  fp_coords : Inport  Port=3
  fp_courses : Inport  Port=4
  Bus Creator1 : BusCreator  Inputs='to_x','to_y','from_x','from_y'
  Course : Subsystem
  From WP : Subsystem
  To WP : Subsystem
  next_leg_course : Outport
  leg_coords : Outport  Port=2
  wires:
  [fp_courses] -> Course/2(fp_courses)
  [fp_coords] -> From WP/2(fp_coords)
  [fp_coords] -> To WP/2(fp_coords)
  fp_courses/1 -> [fp_courses]
  fp_coords/1 -> [fp_coords]
  Course/1(next_leg_crs) -> next_leg_course/1  "next_leg_crs"
  Bus Creator1/1 -> leg_coords/1
  From WP/2(out_y) -> Bus Creator1/4  "from_y"
  From WP/1(out_x) -> Bus Creator1/3  "from_x"
  To WP/2(out_y) -> Bus Creator1/2  "to_y"
  To WP/1(out_x) -> Bus Creator1/1  "to_x"
  to_wp/1 -> Course/1(to wp), To WP/1(to wp)
  from_wp/1 -> From WP/1(to wp)

== system hapsrav_library/Cmd - Parametric/Chi Cmd/Flight Plan/Mission Director/Proximity Distance/Relative Wind ==
  wind_dir : Inport
  chi : Inport  Port=2
  sign : Inport  Port=3
  Product1 : Product
  Sum4 : Sum  Inputs=|+-
  Trigonometric Function2 : Trigonometry
  Trigonometric Function3 : Trigonometry  Operator=cos
  Trigonometric Function4 : Trigonometry  Operator=atan2
  psi_rel : Outport
  wires:
  wind_dir/1 -> Sum4/1
  Trigonometric Function2/1 -> Trigonometric Function4/1
  Sum4/1 -> Trigonometric Function2/1, Trigonometric Function3/1
  Trigonometric Function3/1 -> Trigonometric Function4/2
  chi/1 -> Sum4/2
  Product1/1 -> psi_rel/1
  sign/1 -> Product1/2
  Trigonometric Function4/1 -> Product1/1

== system hapsrav_library/Cmd - Parametric/Chi Cmd/Flight Plan/Mission Director/Proximity Distance/Turn Radius ==
  Vinf : Inport
  Course Change1 : Constant  Value=g
  Course Change2 : Constant  Value=tan_phi_lim
  Divide : Product  Inputs=/*
  Product1 : Product
  Product2 : Product
  rho : Outport
  wires:
  Vinf/1 -> Product1/1, Product1/2
  Divide/1 -> rho/1
  Product1/1 -> Divide/2
  Course Change2/1 -> Product2/1
  Course Change1/1 -> Product2/2
  Product2/1 -> Divide/1

== system hapsrav_library/Cmd - Parametric/Chi Cmd/Subsystem/Figure Eight Orbit/Logic for figure eight following (ready==1) or initialization (ready==0)/Chi Offset (when entering figure eight mode) ==
  chi_cmd : Inport
  ref_axis : Inport  Port=2
  t : Inport  Port=3
  Trigger : TriggerPort  VariantControl=Variant  InitialTriggerSignalState=zero  PortDimensions=1
  chi0_f8 : Outport
  t0_f8 : Outport  Port=2
  ref0_f8 : Outport  Port=3
  wires:
  t/1 -> t0_f8/1
  ref_axis/1 -> ref0_f8/1
  chi_cmd/1 -> chi0_f8/1

== system hapsrav_library/Cmd - Parametric/Chi Cmd/Subsystem/Racetrack Orbit/Pulsing Logic: 1 for hold course 0 for turn/timer ==
  t : Inport
  Trigger : TriggerPort  VariantControl=Variant
  t0 : Outport
  wires:
  t/1 -> t0/1

== system hapsrav_library/hapsrav_main/Kinematic 6DOF/Aero/CL vs AoA/alpha RLUT/0 <= Alt < 20574 ==
  CL : Inport
  alt : Inport  Port=2
  Enable : EnablePort
  1-D Lookup Table : Lookup_n-D  NumberOfTableDimensions=1  BreakpointsForDimension1=cl_data(:,1)  BeginIndexSearchUsingPreviousIndexResult=on  Table=alpha_bp  ExtrapMethod=Clip  RemoveProtectionInput=on  UseLastTableValue=on  InternalRulePriority=Speed  RndMeth=Simplest  InputSameDT=on
  1-D Lookup Table1 : Lookup_n-D  NumberOfTableDimensions=1  BreakpointsForDimension1=cl_data(:,2)  BeginIndexSearchUsingPreviousIndexResult=on  Table=alpha_bp  ExtrapMethod=Clip  RemoveProtectionInput=on  UseLastTableValue=on  InternalRulePriority=Speed  RndMeth=Simplest  InputSameDT=on
  1-D Lookup Table2 : Lookup_n-D  NumberOfTableDimensions=1  BreakpointsForDimension1=alt_bp(1:2)  Table=[1 0]  ExtrapMethod=Clip  RemoveProtectionInput=on  UseLastTableValue=on  InternalRulePriority=Speed  RndMeth=Simplest  InputSameDT=on
  Constant : Constant
  Product : Product
  Product1 : Product
  Sum : Sum  Inputs=|+-
  Sum1 : Sum  Inputs=|++
  alpha : Outport
  wires:
  Sum1/1 -> alpha/1
  Product1/1 -> Sum1/2
  Product/1 -> Sum1/1
  [weight] -> Sum/2
  Sum/1 -> Product1/1
  Constant/1 -> Sum/1
  1-D Lookup Table1/1 -> Product1/2
  [weight] -> Product/1
  1-D Lookup Table/1 -> Product/2
  1-D Lookup Table2/1 -> [weight]
  alt/1 -> 1-D Lookup Table2/1
  CL/1 -> 1-D Lookup Table/1, 1-D Lookup Table1/1

== system hapsrav_library/hapsrav_main/Kinematic 6DOF/Aero/CL vs AoA/alpha RLUT/20574 <= Alt < 21908 ==
  CL : Inport
  alt : Inport  Port=2
  Enable : EnablePort
  1-D Lookup Table : Lookup_n-D  NumberOfTableDimensions=1  BreakpointsForDimension1=cl_data(:,2)  BeginIndexSearchUsingPreviousIndexResult=on  Table=alpha_bp  ExtrapMethod=Clip  RemoveProtectionInput=on  UseLastTableValue=on  InternalRulePriority=Speed  RndMeth=Simplest  InputSameDT=on
  1-D Lookup Table1 : Lookup_n-D  NumberOfTableDimensions=1  BreakpointsForDimension1=cl_data(:,3)  BeginIndexSearchUsingPreviousIndexResult=on  Table=alpha_bp  ExtrapMethod=Clip  RemoveProtectionInput=on  UseLastTableValue=on  InternalRulePriority=Speed  RndMeth=Simplest  InputSameDT=on
  1-D Lookup Table2 : Lookup_n-D  NumberOfTableDimensions=1  BreakpointsForDimension1=alt_bp(2:3)  Table=[1 0]  ExtrapMethod=Clip  RemoveProtectionInput=on  UseLastTableValue=on  InternalRulePriority=Speed  RndMeth=Simplest  InputSameDT=on
  Constant : Constant
  Product : Product
  Product1 : Product
  Sum : Sum  Inputs=|+-
  Sum1 : Sum  Inputs=|++
  alpha : Outport
  wires:
  CL/1 -> 1-D Lookup Table1/1, 1-D Lookup Table/1
  alt/1 -> 1-D Lookup Table2/1
  1-D Lookup Table2/1 -> [weight]
  1-D Lookup Table/1 -> Product/2
  [weight] -> Product/1
  1-D Lookup Table1/1 -> Product1/2
  Constant/1 -> Sum/1
  Sum/1 -> Product1/1
  [weight] -> Sum/2
  Product/1 -> Sum1/1
  Product1/1 -> Sum1/2
  Sum1/1 -> alpha/1

== system hapsrav_library/hapsrav_main/Kinematic 6DOF/Aero/CL vs AoA/alpha RLUT/21908 <= Alt < 23241 ==
  CL : Inport
  alt : Inport  Port=2
  Enable : EnablePort
  1-D Lookup Table : Lookup_n-D  NumberOfTableDimensions=1  BreakpointsForDimension1=cl_data(:,3)  BeginIndexSearchUsingPreviousIndexResult=on  Table=alpha_bp  ExtrapMethod=Clip  RemoveProtectionInput=on  UseLastTableValue=on  InternalRulePriority=Speed  RndMeth=Simplest  InputSameDT=on
  1-D Lookup Table1 : Lookup_n-D  NumberOfTableDimensions=1  BreakpointsForDimension1=cl_data(:,4)  BeginIndexSearchUsingPreviousIndexResult=on  Table=alpha_bp  ExtrapMethod=Clip  RemoveProtectionInput=on  UseLastTableValue=on  InternalRulePriority=Speed  RndMeth=Simplest  InputSameDT=on
  1-D Lookup Table2 : Lookup_n-D  NumberOfTableDimensions=1  BreakpointsForDimension1=alt_bp(3:4)  Table=[1 0]  ExtrapMethod=Clip  RemoveProtectionInput=on  UseLastTableValue=on  InternalRulePriority=Speed  RndMeth=Simplest  InputSameDT=on
  Constant : Constant
  Product : Product
  Product1 : Product
  Sum : Sum  Inputs=|+-
  Sum1 : Sum  Inputs=|++
  alpha : Outport
  wires:
  Sum1/1 -> alpha/1
  Product1/1 -> Sum1/2
  Product/1 -> Sum1/1
  [weight] -> Sum/2
  Sum/1 -> Product1/1
  Constant/1 -> Sum/1
  1-D Lookup Table1/1 -> Product1/2
  [weight] -> Product/1
  1-D Lookup Table/1 -> Product/2
  1-D Lookup Table2/1 -> [weight]
  alt/1 -> 1-D Lookup Table2/1
  CL/1 -> 1-D Lookup Table/1, 1-D Lookup Table1/1

== system hapsrav_library/hapsrav_main/Kinematic 6DOF/Aero/CL vs AoA/alpha RLUT/23241 <= Alt < 24575 ==
  CL : Inport
  alt : Inport  Port=2
  Enable : EnablePort
  1-D Lookup Table : Lookup_n-D  NumberOfTableDimensions=1  BreakpointsForDimension1=cl_data(:,4)  BeginIndexSearchUsingPreviousIndexResult=on  Table=alpha_bp  ExtrapMethod=Clip  RemoveProtectionInput=on  UseLastTableValue=on  InternalRulePriority=Speed  RndMeth=Simplest  InputSameDT=on
  1-D Lookup Table1 : Lookup_n-D  NumberOfTableDimensions=1  BreakpointsForDimension1=cl_data(:,5)  BeginIndexSearchUsingPreviousIndexResult=on  Table=alpha_bp  ExtrapMethod=Clip  RemoveProtectionInput=on  UseLastTableValue=on  InternalRulePriority=Speed  RndMeth=Simplest  InputSameDT=on
  1-D Lookup Table2 : Lookup_n-D  NumberOfTableDimensions=1  BreakpointsForDimension1=alt_bp(4:5)  Table=[1 0]  ExtrapMethod=Clip  RemoveProtectionInput=on  UseLastTableValue=on  InternalRulePriority=Speed  RndMeth=Simplest  InputSameDT=on
  Constant : Constant
  Product : Product
  Product1 : Product
  Sum : Sum  Inputs=|+-
  Sum1 : Sum  Inputs=|++
  alpha : Outport
  wires:
  CL/1 -> 1-D Lookup Table1/1, 1-D Lookup Table/1
  alt/1 -> 1-D Lookup Table2/1
  1-D Lookup Table2/1 -> [weight]
  1-D Lookup Table/1 -> Product/2
  [weight] -> Product/1
  1-D Lookup Table1/1 -> Product1/2
  Constant/1 -> Sum/1
  Sum/1 -> Product1/1
  [weight] -> Sum/2
  Product/1 -> Sum1/1
  Product1/1 -> Sum1/2
  Sum1/1 -> alpha/1

== system hapsrav_library/hapsrav_main/Kinematic 6DOF/Selectable Modes/Trajectory_Optimization/Altitude/alt_rate ==
  max_clmb_rt : Inport
  max_desc_rt : Inport  Port=2
  d2alt : Inport  Port=3
  altRt0 : Inport  Port=4
  idleDesc : Inport  Port=5
  Constant : Constant  Value=dT
  Freezable Limited Integration1 : hapsrav_library/Freezable Limited Integration
  Mux : Mux  Inputs=2
  Scope : Scope
  d1alt : Outport
  wires:
  [dn_lim] -> Freezable Limited Integration1/6
  max_clmb_rt/1 -> [up_lim]
  max_desc_rt/1 -> [dn_lim]
  idleDesc/1 -> Freezable Limited Integration1/4
  altRt0/1 -> Freezable Limited Integration1/3
  [up_lim] -> Freezable Limited Integration1/5
  Constant/1 -> Freezable Limited Integration1/2
  d2alt/1 -> Freezable Limited Integration1/1
  Freezable Limited Integration1/1 -> Mux/1, d1alt/1
  Mux/1 -> Scope/1
  [dn_lim] -> Mux/2

== system hapsrav_library/hapsrav_main/Kinematic 6DOF/Selectable Modes/Trajectory_Optimization/Roll/roll_angle ==
  roll_lim : Inport
  d1roll : Inport  Port=2
  roll0 : Inport  Port=3
  Vg : Inport  Port=4
  chi0 : Inport  Port=5
  Constant : Constant  Value=dT
  Delay1 : Delay  DelayLength=1  InitialConditionSource=Input port
      settings: InputPortMap=u0,p4
  Discrete-Time Integrator : DiscreteIntegrator  IntegratorMethod=Integration: Trapezoidal  InitialConditionSource=external  InitialConditionSetting=State (most efficient)  SampleTime=-1  ICPrevOutput=DiscIntNeverNeededParam  ICPrevScaledInput=DiscIntNeverNeededParam
  Divide : Product  Inputs=*/
  Gain : Gain  Gain=g
  Gain1 : Gain  Gain=-1
  Gain2 : Gain  Gain=1.0
  Limited Integration : MATLAB Function  TreatAsAtomicUnit=on
  Trigonometric Function : Trigonometry  Operator=tan
  chi : Outport
  roll : Outport  Port=2
  wires:
  Gain2/1 -> chi/1
  [roll] -> Trigonometric Function/1
  chi0/1 -> Discrete-Time Integrator/2
  Vg/1 -> Divide/2
  Discrete-Time Integrator/1 -> Gain2/1
  Divide/1 -> Discrete-Time Integrator/1
  Gain/1 -> Divide/1
  Trigonometric Function/1 -> Gain/1
  roll0/1 -> Delay1/2  "roll0"
  Gain1/1 -> Limited Integration/4(lolim)
  roll_lim/1 -> Gain1/1, Limited Integration/3(uplim)
  d1roll/1 -> Limited Integration/1(u)
  Limited Integration/1(y0) -> roll/1, [roll]
  Limited Integration/2(x1) -> Delay1/1
  Delay1/1 -> Limited Integration/5(x0)
  Constant/1 -> Limited Integration/2(T)
